simulink model "modelo_quad13_ver76"  (Simulink 8.3)
settings: Solver=ode45  StartTime=0.0  StopTime=100  FixedStep=0.025  MaxStep=0.1  RelTol=1e-3
values from neighbouring files (symbols this model uses):
  accel_noise = 0    [main_quad.m]
  baccx = 1e-1    (= 0.1)    [main_quad.m]
  baccy = 1e-1    (= 0.1)    [main_quad.m]
  baccz = 1e-1    (= 0.1)    [main_quad.m]
  baro_noise = 0    [main_quad.m]
  bgyrp = 1e-3    (= 0.001)    [main_quad.m]
  bgyrq = 1e-3    (= 0.001)    [main_quad.m]
  bgyrr = 1e-3    (= 0.001)    [main_quad.m]
  bmagx = 1e-6    (= 1e-06)    [main_quad.m]
  bmagy = -1e-6    (= -1e-06)    [main_quad.m]
  bmagz = 1e-6    (= 1e-06)    [main_quad.m]
  controle = 0    [main_quad.m]
  correct_acc = 1    [main_quad.m]
  cq = 2.4086*10^(-7)    (= 2.4086e-07)    [main_quad.m]
  cq_real = cq    (= 2.4086e-07)    [main_quad.m]
  ct = 1.4341*10^(-5)    (= 1.4341e-05)    [main_quad.m]
  ct_real = ct    (= 1.4341e-05)    [main_quad.m]
  d = 0.26    [main_quad.m]
  g = 9.8065    [main_quad.m]
  gps_noise_on = 0    [main_quad.m]
  gyro_noise = 0    [main_quad.m]
  J = [Jxx,Jyy,Jzz,Jm]    [main_quad.m]
  J_real = J    [main_quad.m]
  Ja = 5e-5    (= 5e-05)    [main_quad.m]
  k1 = 2.5    [main_quad.m]
  k2 = 6.2360    (= 6.236)    [main_quad.m]
  k3 = 6.2360    (= 6.236)    [main_quad.m]
  k4 = 0.4927    [main_quad.m]
  k5 = 1.6    [main_quad.m]
  k6 = 1.6    [main_quad.m]
  ke = kt    (= 0.024)    [main_quad.m]
  kt = 0.024    [main_quad.m]
  lambda1 = 1    [main_quad.m]
  lambda2 = 5    [main_quad.m]
  lambda3 = 5    [main_quad.m]
  lambda4 = 1/2    (= 0.5)    [main_quad.m]
  lambda5 = 1/4    (= 0.25)    [main_quad.m]
  lambda6 = 1/4    (= 0.25)    [main_quad.m]
  limit = [0.5 0.5 0.5 0.5]    [main_quad.m]
  limit_pos = [0.5 0.5]    [main_quad.m]
  m = 1.03    [main_quad.m]
  m_real = m    (= 1.03)    [main_quad.m]
  mag_noise = 0    [main_quad.m]
  max_w = 733.03    [main_quad.m]
  mgeo = [17223.7  -4581.6 -13698.2 ]'*1e-9    [main_quad.m]
  p0 = 0    [main_quad.m]
  phi0 = 0    [main_quad.m]
  Pitch_D = 0.019    [main_quad.m]
  Pitch_P = 0.019948    [main_quad.m]
  pos_D = -0.033991    [main_quad.m]
  pos_P = -0.005948    [main_quad.m]
  psi0 = 0    [main_quad.m]
  q0 = 0    [main_quad.m]
  R = 0.2    [main_quad.m]    (also in plot_resultados.m = A(:,12))
  r0 = 0    [main_quad.m]
  Roll_D = 0.019    [main_quad.m]
  Roll_P = 0.019948    [main_quad.m]
  t_d = 50e-3    (= 0.05)    [main_quad.m]
  theta0 = 0    [main_quad.m]
  Tnoise_gps = TsGPS    (= 0.2)    [main_quad.m]
  Ts_bar = 0.1    [main_quad.m]
  TsGPS = 1/fGPS    (= 0.2)    [main_quad.m]
  Tsr = 1e-2    (= 0.01)    [main_quad.m]
  vx0 = 0    [main_quad.m]
  vy0 = 0    [main_quad.m]
  vz0 = 0    [main_quad.m]
  w1_0 = w_hover    [main_quad.m]
  w2_0 = w_hover    [main_quad.m]
  w3_0 = w_hover    [main_quad.m]
  w4_0 = w_hover    [main_quad.m]
  w_f_gps = 2*pi*(2*fGPS)    (= 62.8318530718)    [main_quad.m]
  w_f_triad = 2*pi*(10)    (= 62.8318530718)    [main_quad.m]
  x0 = 0    [main_quad.m]
  y0 = 0    [main_quad.m]
  Yaw_D = 0.037200    (= 0.0372)    [main_quad.m]
  Yaw_P = 0.039055    [main_quad.m]
  z0 = 0    [main_quad.m]
  Z_D = -0.682000    (= -0.682)    [main_quad.m]
  Z_P = -0.238672    [main_quad.m]
libraries: simulink x18
(part 1 of 2)
settings Model: Creator=Germano  LastModifiedBy=andre
settings DataIOCC: LimitDataPoints=off
settings DebuggingCC: FcnCallInpInsideContextMsg=EnableAllAsWarning

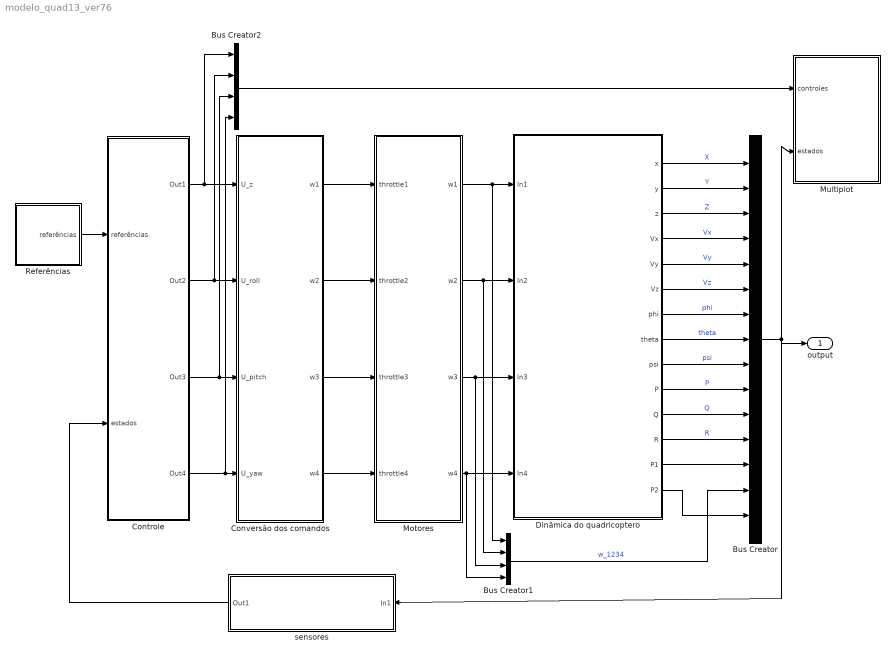
== system modelo_quad13_ver76 ==
  Bus Creator : BusCreator  Inputs=15
  Bus Creator1 : BusCreator
  Bus Creator2 : BusCreator
  Controle : Subsystem
  Conversão dos comandos : Subsystem
  Dinâmica do quadricoptero : Subsystem
  Motores : Subsystem
  Multiplot : Subsystem
  Referências : Subsystem
  sensores : Subsystem
  output : Outport
  wires:
  Bus Creator/1 -> sensores/1(In1), Multiplot/2(estados), output/1
  Motores/4(w4) -> Dinâmica do quadricoptero/4(In4), Bus Creator1/4
  Motores/1(w1) -> Bus Creator1/1, Dinâmica do quadricoptero/1(In1)
  Motores/3(w3) -> Dinâmica do quadricoptero/3(In3), Bus Creator1/3
  Motores/2(w2) -> Bus Creator1/2, Dinâmica do quadricoptero/2(In2)
  Conversão dos comandos/1(w1) -> Motores/1(throttle1)
  Conversão dos comandos/2(w2) -> Motores/2(throttle2)
  Conversão dos comandos/3(w3) -> Motores/3(throttle3)
  Conversão dos comandos/4(w4) -> Motores/4(throttle4)
  Dinâmica do quadricoptero/1(x) -> Bus Creator/1  "X"
  Dinâmica do quadricoptero/2(y) -> Bus Creator/2  "Y"
  Dinâmica do quadricoptero/3(z) -> Bus Creator/3  "Z"
  Dinâmica do quadricoptero/4(Vx) -> Bus Creator/4  "Vx"
  Dinâmica do quadricoptero/5(Vy) -> Bus Creator/5  "Vy"
  Dinâmica do quadricoptero/6(Vz) -> Bus Creator/6  "Vz"
  Dinâmica do quadricoptero/7(phi) -> Bus Creator/7  "phi"
  Dinâmica do quadricoptero/8(theta) -> Bus Creator/8  "theta"
  Dinâmica do quadricoptero/9(psi) -> Bus Creator/9  "psi"
  Dinâmica do quadricoptero/10(P) -> Bus Creator/10  "P"
  Dinâmica do quadricoptero/11(Q) -> Bus Creator/11  "Q"
  Dinâmica do quadricoptero/12(R) -> Bus Creator/12  "R"
  Controle/1(Out1) -> Bus Creator2/1, Conversão dos comandos/1(U_z)
  Controle/2(Out2) -> Bus Creator2/2, Conversão dos comandos/2(U_roll)
  Controle/3(Out3) -> Bus Creator2/3, Conversão dos comandos/3(U_pitch)
  Controle/4(Out4) -> Bus Creator2/4, Conversão dos comandos/4(U_yaw)
  Referências/1("referências ") -> Controle/1(referências)
  sensores/1(Out1) -> Controle/2(estados)
  Bus Creator2/1 -> Multiplot/1(controles)
  Dinâmica do quadricoptero/13(P1) -> Bus Creator/13
  Bus Creator1/1 -> Bus Creator/14  "w_1234"
  Dinâmica do quadricoptero/14(P2) -> Bus Creator/15

== system modelo_quad13_ver76/Controle ==
  note: 0: controle Sliding Mode
      | 1: controle PD
  referências : Inport
  estados : Inport  Port=2
  Constant : Constant  Value=controle
  Controlador PD : Subsystem
  Controlador sliding mode : Subsystem
  Demux : Demux
  Switch : Switch  Criteria=u2 > Threshold
  Out1 : Outport
  Out2 : Outport  Port=2
  Out3 : Outport  Port=3
  Out4 : Outport  Port=4
  wires:
  referências/1 -> Controlador sliding mode/1(Referências), Controlador PD/1(Referências)
  estados/1 -> Controlador sliding mode/2(Estados), Controlador PD/2(Estados)
  Switch/1 -> Demux/1
  Demux/1 -> Out1/1  "U_T"
  Demux/2 -> Out2/1  "U_L"
  Constant/1 -> Switch/2
  Demux/3 -> Out3/1  "U_M"
  Demux/4 -> Out4/1  "U_N"
  Controlador PD/1(Out1) -> Switch/1
  Controlador sliding mode/1(Out1) -> Switch/3

== system modelo_quad13_ver76/Conversão dos comandos ==
  U_z : Inport
  U_roll : Inport  Port=2
  U_pitch : Inport  Port=3
  U_yaw : Inport  Port=4
  Constant1 : Constant  Value=ct
  Constant2 : Constant  Value=cq
  Constant4 : Constant  Value=d
  MATLAB Function : MATLAB Function  TreatAsAtomicUnit=on
  w1 : Outport
  w2 : Outport  Port=2
  w3 : Outport  Port=3
  w4 : Outport  Port=4
  wires:
  U_pitch/1 -> MATLAB Function/3(u_M)
  U_z/1 -> MATLAB Function/1(u_T)
  U_yaw/1 -> MATLAB Function/4(u_N)
  Constant4/1 -> MATLAB Function/5(d)
  Constant1/1 -> MATLAB Function/6(ct)
  Constant2/1 -> MATLAB Function/7(cq)
  U_roll/1 -> MATLAB Function/2(u_L)
  MATLAB Function/1(w1d) -> w1/1  "w1d"
  MATLAB Function/2(w2d) -> w2/1  "w2d"
  MATLAB Function/3(w3d) -> w3/1  "w3d"
  MATLAB Function/4(w4d) -> w4/1  "w4d"

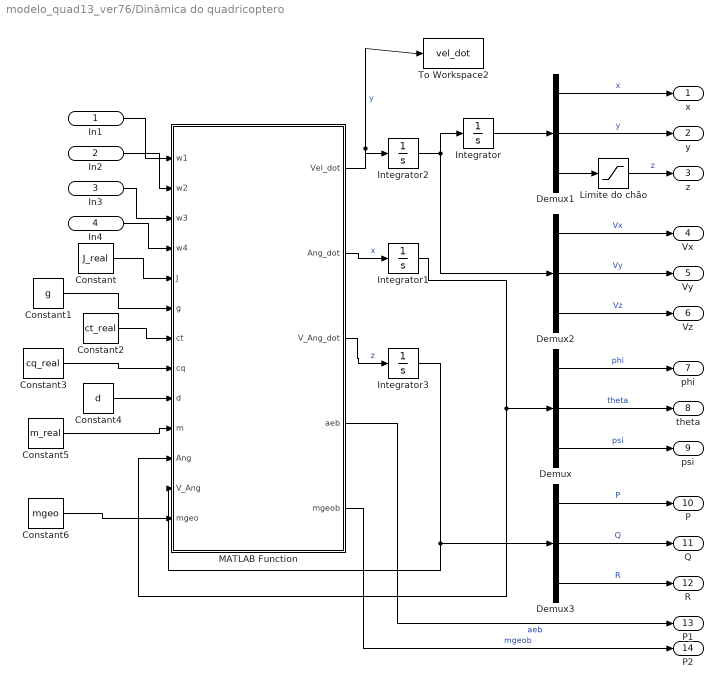
== system modelo_quad13_ver76/Dinâmica do quadricoptero ==
  In1 : Inport
  In2 : Inport  Port=2
  In3 : Inport  Port=3
  In4 : Inport  Port=4
  Constant : Constant  Value=J_real
  Constant1 : Constant  Value=g
  Constant2 : Constant  Value=ct_real
  Constant3 : Constant  Value=cq_real
  Constant4 : Constant  Value=d
  Constant5 : Constant  Value=m_real
  Constant6 : Constant  Value=mgeo
  Demux{,1..3} (4 alike) : Demux  Outputs=3
  Integrator : Integrator  InitialCondition=[x0;y0;z0]
  Integrator1 : Integrator  InitialCondition=[phi0;theta0;psi0]
  Integrator2 : Integrator  InitialCondition=[vx0;vy0;vz0;]
  Integrator3 : Integrator  InitialCondition=[p0;q0;r0]
  Limite do chão : Saturate  UpperLimit=0  LowerLimit=-Inf
  MATLAB Function : MATLAB Function  TreatAsAtomicUnit=on
  To Workspace2 : ToWorkspace  VariableName=vel_dot  SampleTime=-1
  x : Outport
  y : Outport  Port=2
  z : Outport  Port=3
  Vx : Outport  Port=4
  Vy : Outport  Port=5
  Vz : Outport  Port=6
  phi : Outport  Port=7
  theta : Outport  Port=8
  psi : Outport  Port=9
  P : Outport  Port=10
  Q : Outport  Port=11
  R : Outport  Port=12
  P1 : Outport  Port=13
  P2 : Outport  Port=14
  wires:
  In1/1 -> MATLAB Function/1(w1)
  In2/1 -> MATLAB Function/2(w2)
  In3/1 -> MATLAB Function/3(w3)
  In4/1 -> MATLAB Function/4(w4)
  Demux1/1 -> x/1  "x"
  Demux1/2 -> y/1  "y"
  Demux2/1 -> Vx/1  "Vx"
  Demux2/2 -> Vy/1  "Vy"
  Demux2/3 -> Vz/1  "Vz"
  MATLAB Function/1(Vel_dot) -> To Workspace2/1, Integrator2/1  "y"
  Integrator1/1 -> Demux/1, MATLAB Function/11(Ang)
  Demux/1 -> phi/1  "phi"
  Demux/2 -> theta/1  "theta"
  Demux/3 -> psi/1  "psi"
  MATLAB Function/2(Ang_dot) -> Integrator1/1  "x"
  Demux3/1 -> P/1  "P"
  Demux3/2 -> Q/1  "Q"
  Demux3/3 -> R/1  "R"
  MATLAB Function/3(V_Ang_dot) -> Integrator3/1  "z"
  Integrator2/1 -> Demux2/1, Integrator/1
  Integrator3/1 -> Demux3/1, MATLAB Function/12(V_Ang)
  Constant/1 -> MATLAB Function/5(J)
  Constant1/1 -> MATLAB Function/6(g)
  Constant2/1 -> MATLAB Function/7(ct)
  Constant3/1 -> MATLAB Function/8(cq)
  Constant4/1 -> MATLAB Function/9(d)
  Constant5/1 -> MATLAB Function/10(m)
  Integrator/1 -> Demux1/1
  Demux1/3 -> Limite do chão/1
  Limite do chão/1 -> z/1  "z"
  MATLAB Function/4(aeb) -> P1/1  "aeb"
  MATLAB Function/5(mgeob) -> P2/1  "mgeob"
  Constant6/1 -> MATLAB Function/13(mgeo)

== system modelo_quad13_ver76/Motores ==
  throttle1 : Inport
  throttle2 : Inport  Port=2
  throttle3 : Inport  Port=3
  throttle4 : Inport  Port=4
  Motor 1 : Subsystem
  Motor 2 : Subsystem
  Motor 3 : Subsystem
  Motor 4 : Subsystem
  w1 : Outport
  w2 : Outport  Port=2
  w3 : Outport  Port=3
  w4 : Outport  Port=4
  wires:
  throttle1/1 -> Motor 1/1(In1)  "w1d"
  throttle3/1 -> Motor 3/1(In1)  "w3d"
  throttle4/1 -> Motor 4/1(In1)  "w4d"
  throttle2/1 -> Motor 2/1(In1)  "w2d"
  Motor 1/1(Out1) -> w1/1  "w1"
  Motor 3/1(Out1) -> w3/1  "w3"
  Motor 4/1(Out1) -> w4/1  "w4"
  Motor 2/1(Out1) -> w2/1  "w2"

== system modelo_quad13_ver76/Multiplot ==
  controles : Inport
  estados : Inport  Port=2
  Bus Creator{1..4} (4 alike) : BusCreator  Inputs=3
  Bus Selector : BusSelector  OutputSignals=X,Y,Z,Vx,Vy,Vz,phi,theta,psi,P,Q,R,w_1234
  Gain : Gain  Gain=-1
  Gain1 : Gain  Gain=-1
  Gain2 : Gain  Gain=180/pi
  Gain3 : Gain  Gain=180/pi
  Gain4 : Gain  Gain=9.54929
  wires:
  estados/1 -> Bus Selector/1
  Bus Selector/2 -> Bus Creator2/2  "<Y>"
  Bus Selector/3 -> Gain/1  "<Z>"
  Bus Selector/1 -> Bus Creator2/1  "<X>"
  Bus Selector/6 -> Gain1/1  "<Vz>"
  Bus Selector/4 -> Bus Creator1/1  "<Vx>"
  Bus Selector/5 -> Bus Creator1/2  "<Vy>"
  Bus Selector/8 -> Bus Creator3/2  "<theta>"
  Bus Selector/7 -> Bus Creator3/1  "<phi>"
  Bus Selector/9 -> Bus Creator3/3  "<psi>"
  Bus Selector/11 -> Bus Creator4/2  "<Q>"
  Bus Selector/10 -> Bus Creator4/1  "<P>"
  Bus Selector/12 -> Bus Creator4/3  "<R>"
  Bus Creator2/1 -> ?
  Bus Creator1/1 -> ?
  controles/1 -> ?
  Gain/1 -> Bus Creator2/3
  Gain1/1 -> Bus Creator1/3
  Bus Creator3/1 -> Gain2/1
  Gain2/1 -> ?
  Bus Creator4/1 -> Gain3/1
  Gain3/1 -> ?
  Bus Selector/13 -> Gain4/1  "<w_1234>"
  Gain4/1 -> ?

== system modelo_quad13_ver76/Referências ==
  Gain1 : Gain
  Gain2 : Gain
  Gain3 : Gain  Gain=-1
  Gain4 : Gain
  Mux : Mux
  Step1 : Step  Time=75  After=15*pi/180  SampleTime=0
  Step2 : Step  Time=5  After=10  SampleTime=0
  Step_x : Step  Time=10  After=10  SampleTime=0
  Step_y : Step  Time=30  After=10  SampleTime=0
  "referências " : Outport
  wires:
  Mux/1 -> "referências "/1
  Gain3/1 -> Mux/3  "ref_z"
  Step_y/1 -> Gain2/1
  Gain2/1 -> Mux/2  "ref_y"
  Step_x/1 -> Gain4/1
  Gain4/1 -> Mux/1  "ref_x"
  Gain1/1 -> Mux/4  "ref_psi"
  Step2/1 -> Gain3/1
  Step1/1 -> Gain1/1

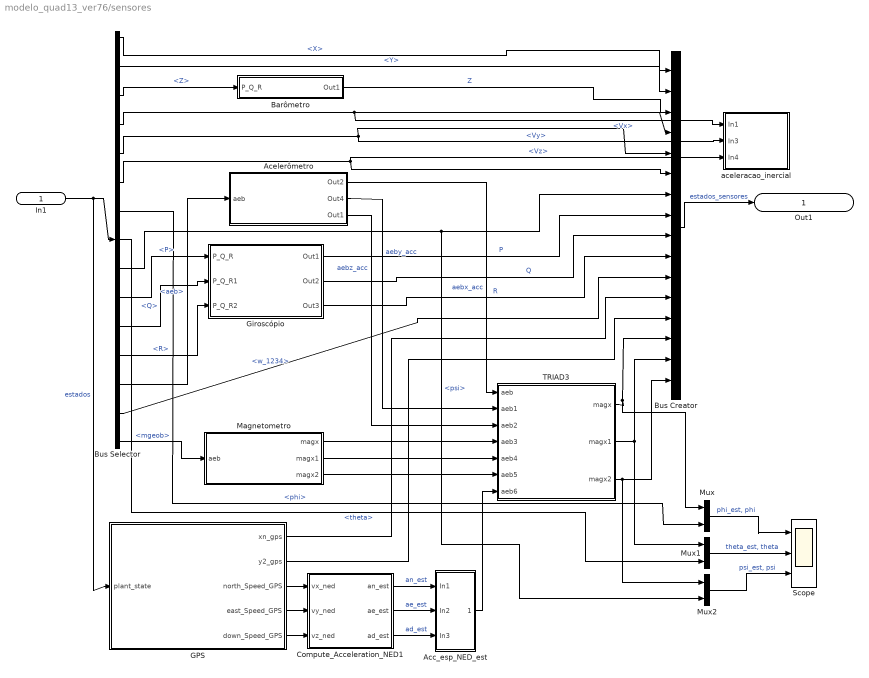
== system modelo_quad13_ver76/sensores ==
  In1 : Inport
  Acc_esp_NED_est : Subsystem
  Acelerômetro : Subsystem
  Barômetro : Subsystem
  Bus Creator : BusCreator  Inputs=16
  Bus Selector : BusSelector  OutputSignals=X,Y,Z,Vx,Vy,Vz,phi,theta,psi,P,Q,R,aeb,w_1234,mgeob
  Compute_Acceleration_NED1 : Subsystem
  GPS : Subsystem
  Giroscópio : Subsystem
  Magnetometro : Subsystem
  Mux : Mux  Inputs=2
  Mux1 : Mux  Inputs=2
  Mux2 : Mux  Inputs=2
  Scope : Scope  NumInputPorts=3
      settings: YMin=-2.5~-1.5~-1.75  YMax=2~0.25~1.75  SaveName=ScopeData8
  TRIAD3 : Subsystem
  aceleracao_inercial : Subsystem
  Out1 : Outport
  wires:
  In1/1 -> Bus Selector/1, GPS/1(plant_state)  "estados"
  Bus Selector/4 -> Bus Creator/4, aceleracao_inercial/1(In1)  "<Vx>"
  Bus Selector/6 -> Bus Creator/6, aceleracao_inercial/3(In4)  "<Vz>"
  Bus Selector/1 -> Bus Creator/1  "<X>"
  Bus Selector/3 -> Barômetro/1(P_Q_R)  "<Z>"
  Bus Selector/2 -> Bus Creator/2  "<Y>"
  Bus Selector/5 -> Bus Creator/5, aceleracao_inercial/2(In3)  "<Vy>"
  Bus Creator/1 -> Out1/1  "estados_sensores"
  Bus Selector/10 -> Giroscópio/1(P_Q_R)  "<P>"
  Bus Selector/11 -> Giroscópio/2(P_Q_R1)  "<Q>"
  Bus Selector/12 -> Giroscópio/3(P_Q_R2)  "<R>"
  Giroscópio/3(Out3) -> Bus Creator/10  "R"
  Giroscópio/2(Out2) -> Bus Creator/9  "Q"
  Giroscópio/1(Out1) -> Bus Creator/8  "P"
  Bus Selector/14 -> Bus Creator/11  "<w_1234>"
  Bus Selector/9 -> Bus Creator/7, Mux2/2  "<psi>"
  Bus Selector/13 -> Acelerômetro/1(aeb)  "<aeb>"
  Bus Selector/15 -> Magnetometro/1(aeb)  "<mgeob>"
  Acelerômetro/1(Out2) -> TRIAD3/1(aeb)  "aebx_acc"
  Acelerômetro/2(Out4) -> TRIAD3/2(aeb1)  "aeby_acc"
  Acelerômetro/3(Out1) -> TRIAD3/3(aeb2)  "aebz_acc"
  Magnetometro/1(magx) -> TRIAD3/4(aeb3)
  Magnetometro/2(magx1) -> TRIAD3/5(aeb4)
  Magnetometro/3(magx2) -> TRIAD3/6(aeb5)
  GPS/2(y2_gps) -> Bus Creator/13
  GPS/3(north_Speed_GPS) -> Compute_Acceleration_NED1/1(vx_ned)
  GPS/4(east_Speed_GPS) -> Compute_Acceleration_NED1/2(vy_ned)
  GPS/5(down_Speed_GPS) -> Compute_Acceleration_NED1/3(vz_ned)
  Compute_Acceleration_NED1/1(an_est) -> Acc_esp_NED_est/1(In1)  "an_est"
  Compute_Acceleration_NED1/2(ae_est) -> Acc_esp_NED_est/2(In2)  "ae_est"
  Compute_Acceleration_NED1/3(ad_est) -> Acc_esp_NED_est/3(In3)  "ad_est"
  Acc_esp_NED_est/1(Out1) -> TRIAD3/7(aeb6)
  GPS/1(xn_gps) -> Bus Creator/12
  Barômetro/1(Out1) -> Bus Creator/3  "Z"
  TRIAD3/1(magx) -> Bus Creator/14, Mux/1
  TRIAD3/2(magx1) -> Bus Creator/15, Mux1/1
  TRIAD3/3(magx2) -> Bus Creator/16, Mux2/1
  Mux/1 -> Scope/1  "phi_est, phi"
  Mux1/1 -> Scope/2  "theta_est, theta"
  Mux2/1 -> Scope/3  "psi_est, psi"
  Bus Selector/8 -> Mux1/2  "<theta>"
  Bus Selector/7 -> Mux/2  "<phi>"

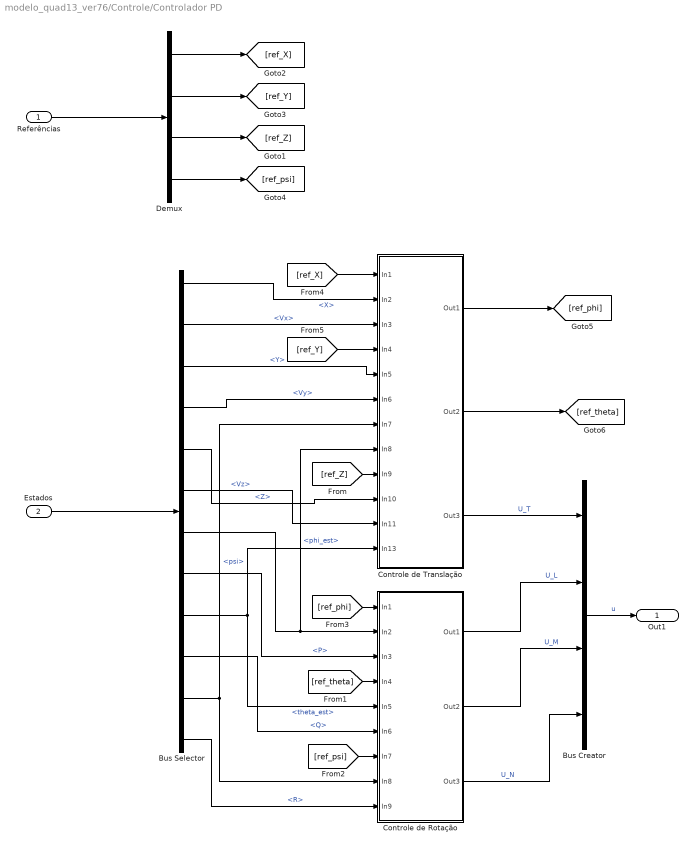
== system modelo_quad13_ver76/Controle/Controlador PD ==
  Referências : Inport
  Estados : Inport  Port=2
  Bus Creator : BusCreator
  Bus Selector : BusSelector  OutputSignals=X,Vx,Y,Vy,Z,Vz,phi_est,P,theta_est,Q,psi,R
  Controle de Rotação : Subsystem
  Controle de Translação : Subsystem
  Demux : Demux
  Out1 : Outport
  wires:
  Demux/4 -> [ref_psi]
  Bus Creator/1 -> Out1/1  "u"
  Demux/1 -> [ref_X]
  Demux/2 -> [ref_Y]
  Demux/3 -> [ref_Z]
  [ref_phi] -> Controle de Rotação/1(In1)
  [ref_theta] -> Controle de Rotação/4(In4)
  Controle de Rotação/1(Out1) -> Bus Creator/2  "U_L"
  Controle de Rotação/2(Out2) -> Bus Creator/3  "U_M"
  Controle de Rotação/3(Out3) -> Bus Creator/4  "U_N"
  [ref_X] -> Controle de Translação/1(In1)
  Controle de Translação/3(Out3) -> Bus Creator/1  "U_T"
  [ref_Y] -> Controle de Translação/4(In4)
  [ref_Z] -> Controle de Translação/9(In9)
  Bus Selector/1 -> Controle de Translação/2(In2)  "<X>"
  Bus Selector/2 -> Controle de Translação/3(In3)  "<Vx>"
  Bus Selector/3 -> Controle de Translação/5(In5)  "<Y>"
  Bus Selector/4 -> Controle de Translação/6(In6)  "<Vy>"
  Bus Selector/5 -> Controle de Translação/10(In10)  "<Z>"
  Bus Selector/6 -> Controle de Translação/11(In11)  "<Vz>"
  Bus Selector/7 -> Controle de Translação/8(In8), Controle de Rotação/2(In2)  "<phi_est>"
  Bus Selector/8 -> Controle de Rotação/3(In3)  "<P>"
  Bus Selector/9 -> Controle de Rotação/5(In5), Controle de Translação/12(In13)  "<theta_est>"
  Bus Selector/10 -> Controle de Rotação/6(In6)  "<Q>"
  Bus Selector/11 -> Controle de Rotação/8(In8), Controle de Translação/7(In7)  "<psi>"
  Bus Selector/12 -> Controle de Rotação/9(In9)  "<R>"
  [ref_psi] -> Controle de Rotação/7(In7)
  Referências/1 -> Demux/1
  Estados/1 -> Bus Selector/1
  Controle de Translação/1(Out1) -> [ref_phi]
  Controle de Translação/2(Out2) -> [ref_theta]

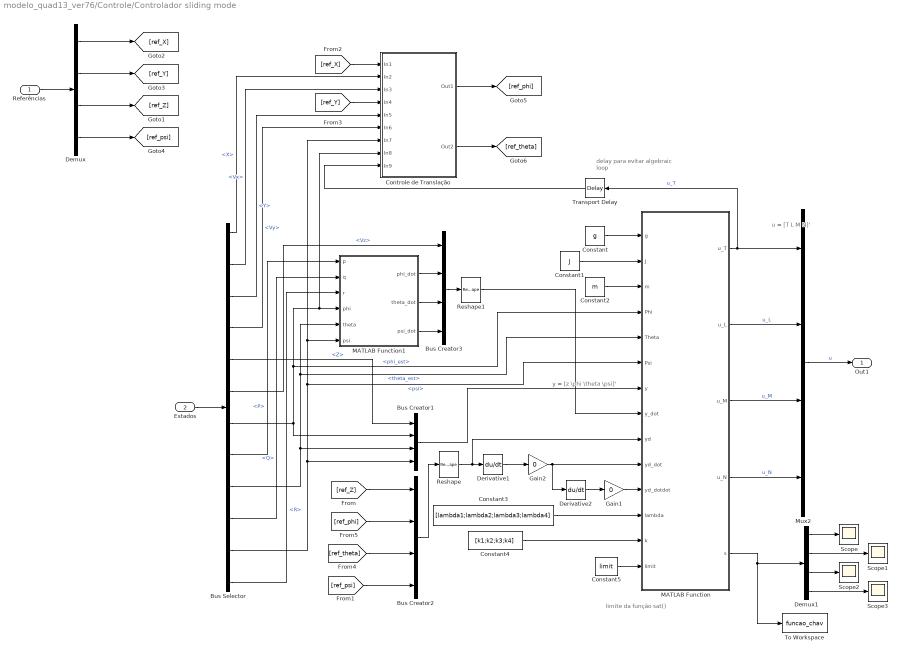
== system modelo_quad13_ver76/Controle/Controlador sliding mode ==
  note: limite da função sat()
  note: delay para evitar
      |  algebraic loop
  note: y = [z \phi \theta \psi]'
  note: u = [T L M N]'
  Referências : Inport
  Estados : Inport  Port=2
  Bus Creator1 : BusCreator
  Bus Creator2 : BusCreator
  Bus Creator3 : BusCreator
  Bus Selector : BusSelector  OutputSignals=X,Vx,Y,Vy,Z,Vz,phi_est,P,theta_est,Q,psi,R
  Constant : Constant  Value=g
  Constant1 : Constant  Value=J
  Constant2 : Constant  Value=m
  Constant3 : Constant  Value=[lambda1;lambda2;lambda3;lambda4]
  Constant4 : Constant  Value=[k1;k2;k3;k4]
  Constant5 : Constant  Value=limit
  Controle de Translação : Subsystem
  Demux : Demux
  Demux1 : Demux
  Derivative1 : Derivative
  Derivative2 : Derivative
  Gain1 : Gain  Gain=0
  Gain2 : Gain  Gain=0
  MATLAB Function : MATLAB Function  TreatAsAtomicUnit=on
  MATLAB Function1 : MATLAB Function  TreatAsAtomicUnit=on
  Mux2 : Mux
  Reshape : Reshape  OutputDimensionality=Customize  OutputDimensions=[4,1]
  Reshape1 : Reshape  OutputDimensionality=Customize  OutputDimensions=[4,1]
  Scope{,1..3} (4 alike) : Scope
      Scope settings: TimeRange=100  YMin=-1
      Scope1 settings: TimeRange=100  YMin=-1  SaveName=ScopeData4
      Scope2 settings: TimeRange=100  YMin=-1  SaveName=ScopeData5
      Scope3 settings: TimeRange=100  YMin=-1  SaveName=ScopeData6
  To Workspace : ToWorkspace  VariableName=funcao_chav  SampleTime=-1
  Transport Delay : TransportDelay  DelayTime=0.01  InitialOutput=m*g
  Out1 : Outport
  wires:
  Demux/4 -> [ref_psi]
  Estados/1 -> Bus Selector/1
  Referências/1 -> Demux/1
  Demux/1 -> [ref_X]
  Demux/2 -> [ref_Y]
  Demux/3 -> [ref_Z]
  Constant/1 -> MATLAB Function/1(g)
  Constant1/1 -> MATLAB Function/2(J)
  Constant2/1 -> MATLAB Function/3(m)
  Bus Selector/5 -> Bus Creator1/1  "<Z>"
  Bus Selector/7 -> Bus Creator1/2, MATLAB Function/4(Phi), Controle de Translação/8(In8), MATLAB Function1/4(phi)  "<phi_est>"
  Bus Selector/9 -> Bus Creator1/3, MATLAB Function/5(Theta), MATLAB Function1/5(theta)  "<theta_est>"
  Bus Selector/11 -> Bus Creator1/4, Controle de Translação/7(In7), MATLAB Function1/6(psi), MATLAB Function/6(Psi)  "<psi>"
  Constant3/1 -> MATLAB Function/12(lambda)
  Bus Selector/8 -> MATLAB Function1/1(p)  "<P>"
  Bus Selector/10 -> MATLAB Function1/2(q)  "<Q>"
  Bus Selector/12 -> MATLAB Function1/3(r)  "<R>"
  Constant4/1 -> MATLAB Function/13(k)
  Derivative2/1 -> Gain1/1
  Mux2/1 -> Out1/1  "u"
  MATLAB Function/1(u_T) -> Mux2/1, Transport Delay/1  "u_T"
  MATLAB Function/2(u_L) -> Mux2/2  "u_L"
  MATLAB Function/4(u_N) -> Mux2/4  "u_N"
  MATLAB Function/3(u_M) -> Mux2/3  "u_M"
  Gain1/1 -> MATLAB Function/11(yd_dotdot)
  Gain2/1 -> Derivative2/1, MATLAB Function/10(yd_dot)
  Bus Selector/1 -> Controle de Translação/2(In2)  "<X>"
  Bus Selector/2 -> Controle de Translação/3(In3)  "<Vx>"
  Bus Selector/3 -> Controle de Translação/5(In5)  "<Y>"
  Bus Selector/4 -> Controle de Translação/6(In6)  "<Vy>"
  [ref_X] -> Controle de Translação/1(In1)
  [ref_Y] -> Controle de Translação/4(In4)
  [ref_Z] -> Bus Creator2/1
  [ref_psi] -> Bus Creator2/4
  Bus Creator2/1 -> Reshape/1
  [ref_theta] -> Bus Creator2/3
  [ref_phi] -> Bus Creator2/2
  Bus Creator1/1 -> MATLAB Function/7(y)
  Controle de Translação/1(Out1) -> [ref_phi]
  Controle de Translação/2(Out2) -> [ref_theta]
  Reshape/1 -> MATLAB Function/9(yd), Derivative1/1
  Transport Delay/1 -> Controle de Translação/9(In9)
  Constant5/1 -> MATLAB Function/14(limit)
  Bus Selector/6 -> Bus Creator3/1  "<Vz>"
  MATLAB Function1/1(phi_dot) -> Bus Creator3/2
  MATLAB Function1/2(theta_dot) -> Bus Creator3/3
  MATLAB Function1/3(psi_dot) -> Bus Creator3/4
  Bus Creator3/1 -> Reshape1/1
  Reshape1/1 -> MATLAB Function/8(y_dot)
  MATLAB Function/5(s) -> Demux1/1, To Workspace/1
  Derivative1/1 -> Gain2/1
  Demux1/1 -> Scope/1
  Demux1/2 -> Scope1/1
  Demux1/3 -> Scope2/1
  Demux1/4 -> Scope3/1

== system modelo_quad13_ver76/Motores/Motor 1 ==
  In1 : Inport
  Constant : Constant  Value=ke
  Constant1 : Constant  Value=cq
  Constant2 : Constant  Value=kt
  Constant3 : Constant  Value=R
  Constant4 : Constant  Value=Ja
  Integrator : Integrator  InitialCondition=w1_0
  MATLAB Function : MATLAB Function  TreatAsAtomicUnit=on
  Saturation : Saturate  UpperLimit=max_w  LowerLimit=0
  Out1 : Outport
  wires:
  MATLAB Function/1(wder) -> Integrator/1
  Saturation/1 -> MATLAB Function/2(w), Out1/1  "w1"
  Integrator/1 -> Saturation/1
  Constant/1 -> MATLAB Function/3(ke)
  Constant1/1 -> MATLAB Function/4(cq)
  Constant2/1 -> MATLAB Function/5(kt)
  Constant3/1 -> MATLAB Function/6(R)
  Constant4/1 -> MATLAB Function/7(Ja)
  In1/1 -> MATLAB Function/1(wd)

== system modelo_quad13_ver76/Motores/Motor 2 ==
  In1 : Inport
  Constant : Constant  Value=ke
  Constant1 : Constant  Value=cq
  Constant2 : Constant  Value=kt
  Constant3 : Constant  Value=R
  Constant4 : Constant  Value=Ja
  Integrator : Integrator  InitialCondition=w2_0
  MATLAB Function : MATLAB Function  TreatAsAtomicUnit=on
  Saturation : Saturate  UpperLimit=max_w  LowerLimit=0
  Out1 : Outport
  wires:
  MATLAB Function/1(wder) -> Integrator/1
  Saturation/1 -> MATLAB Function/2(w), Out1/1  "w2"
  Integrator/1 -> Saturation/1
  Constant/1 -> MATLAB Function/3(ke)
  Constant1/1 -> MATLAB Function/4(cq)
  Constant2/1 -> MATLAB Function/5(kt)
  Constant3/1 -> MATLAB Function/6(R)
  Constant4/1 -> MATLAB Function/7(Ja)
  In1/1 -> MATLAB Function/1(wd)

== system modelo_quad13_ver76/Motores/Motor 3 ==
  In1 : Inport
  Constant : Constant  Value=ke
  Constant1 : Constant  Value=cq
  Constant2 : Constant  Value=kt
  Constant3 : Constant  Value=R
  Constant4 : Constant  Value=Ja
  Integrator : Integrator  InitialCondition=w3_0
  MATLAB Function : MATLAB Function  TreatAsAtomicUnit=on
  Saturation : Saturate  UpperLimit=max_w  LowerLimit=0
  Out1 : Outport
  wires:
  MATLAB Function/1(wder) -> Integrator/1
  Saturation/1 -> MATLAB Function/2(w), Out1/1  "w3"
  Integrator/1 -> Saturation/1
  Constant/1 -> MATLAB Function/3(ke)
  Constant1/1 -> MATLAB Function/4(cq)
  Constant2/1 -> MATLAB Function/5(kt)
  Constant3/1 -> MATLAB Function/6(R)
  Constant4/1 -> MATLAB Function/7(Ja)
  In1/1 -> MATLAB Function/1(wd)

== system modelo_quad13_ver76/Motores/Motor 4 ==
  In1 : Inport
  Constant : Constant  Value=ke
  Constant1 : Constant  Value=cq
  Constant2 : Constant  Value=kt
  Constant3 : Constant  Value=R
  Constant4 : Constant  Value=Ja
  Integrator : Integrator  InitialCondition=w4_0
  MATLAB Function : MATLAB Function  TreatAsAtomicUnit=on
  Saturation : Saturate  UpperLimit=max_w  LowerLimit=0
  Out1 : Outport
  wires:
  MATLAB Function/1(wder) -> Integrator/1
  Saturation/1 -> MATLAB Function/2(w), Out1/1  "w4"
  Integrator/1 -> Saturation/1
  Constant/1 -> MATLAB Function/3(ke)
  Constant1/1 -> MATLAB Function/4(cq)
  Constant2/1 -> MATLAB Function/5(kt)
  Constant3/1 -> MATLAB Function/6(R)
  Constant4/1 -> MATLAB Function/7(Ja)
  In1/1 -> MATLAB Function/1(wd)

== system modelo_quad13_ver76/sensores/Acc_esp_NED_est ==
  In1 : Inport
  In2 : Inport  Port=2
  In3 : Inport  Port=3
  Add : Sum  Inputs=+-
  Gain : Gain  Gain=correct_acc
  Mux2 : Mux  Inputs=3
  acc_grav_ned : Constant  Value=[0 0 g]'
  Out1 : Outport
  wires:
  Mux2/1 -> Gain/1  "acc_ned_est"
  acc_grav_ned/1 -> Add/2
  In1/1 -> Mux2/1  "an_ned"
  In2/1 -> Mux2/2  "ae_ned"
  Add/1 -> Out1/1  "a_esp_ned"
  In3/1 -> Mux2/3  "ad_ned"
  Gain/1 -> Add/1

== system modelo_quad13_ver76/sensores/Acelerômetro ==
  aeb : Inport
  Demux : Demux  Outputs=3
  Inclusão ruídos : Subsystem
  Scope1 : Scope  NumInputPorts=3
      settings: YMin=-0.75~-0.75~-10.75  YMax=1~1~-8.75  SaveName=ScopeData9
  Out2 : Outport
  Out4 : Outport  Port=2
  Out1 : Outport  Port=3
  wires:
  aeb/1 -> Demux/1  "aeb"
  Demux/2 -> Inclusão ruídos/2(P_Q_R1)
  Demux/3 -> Inclusão ruídos/3(P_Q_R2)
  Demux/1 -> Inclusão ruídos/1(P_Q_R)
  Inclusão ruídos/1(Out1) -> Out2/1, Scope1/1  "aebx_acc"
  Inclusão ruídos/2(Out2) -> Out4/1, Scope1/2  "aeby_acc"
  Inclusão ruídos/3(Out3) -> Out1/1, Scope1/3  "aebz_acc"

== system modelo_quad13_ver76/sensores/Barômetro ==
  P_Q_R : Inport
  Add3 : Sum
  Band-Limited White Noise : simulink/Sources/Band-Limited White Noise  Cov=varbar  Ts=Ts_bar  seed=[23341]
  Gain : Gain  Gain=baro_noise
  Scope : Scope
      settings: YMin=-13  YMax=3  SaveName=ScopeData12
  Out1 : Outport
  wires:
  Add3/1 -> Out1/1, Scope/1  "z_baro"
  P_Q_R/1 -> Add3/1  "z"
  Band-Limited White Noise/1 -> Gain/1
  Gain/1 -> Add3/2

== system modelo_quad13_ver76/sensores/Compute_Acceleration_NED1 ==
  vx_ned : Inport
  vy_ned : Inport  Port=2
  vz_ned : Inport  Port=3
  Scope : Scope  NumInputPorts=3
      settings: YMin=-1~-1~-2.5  YMax=1~1~0
  Scope1 : Scope  NumInputPorts=3
      settings: YMin=-50~-75~-125  YMax=50~75~100  SaveName=ScopeData2
  Transfer Fcn : TransferFcn  Numerator=[1 0]  Denominator=[t_d 1]
  Transfer Fcn1 : TransferFcn  Numerator=[1 0]  Denominator=[t_d 1]
  Transfer Fcn2 : TransferFcn  Numerator=[1 0]  Denominator=[t_d 1]
  Transfer Fcn3 : TransferFcn  Numerator=[w_f_gps]  Denominator=[1 w_f_gps]
  Transfer Fcn4 : TransferFcn  Numerator=[w_f_gps]  Denominator=[1 w_f_gps]
  Transfer Fcn5 : TransferFcn  Numerator=[w_f_gps]  Denominator=[1 w_f_gps]
  an_est : Outport
  ae_est : Outport  Port=2
  ad_est : Outport  Port=3
  wires:
  vy_ned/1 -> Transfer Fcn4/1
  vx_ned/1 -> Transfer Fcn3/1
  vz_ned/1 -> Transfer Fcn5/1
  Transfer Fcn/1 -> an_est/1, Scope1/1
  Transfer Fcn1/1 -> ae_est/1, Scope1/2
  Transfer Fcn2/1 -> ad_est/1, Scope1/3
  Transfer Fcn3/1 -> Scope/1, Transfer Fcn/1
  Transfer Fcn4/1 -> Scope/2, Transfer Fcn1/1
  Transfer Fcn5/1 -> Scope/3, Transfer Fcn2/1

== system modelo_quad13_ver76/sensores/GPS ==
  plant_state : Inport
  Bus Selector : BusSelector  OutputSignals=X,Y,Vx,Vy,Vz
  GPS_LAT : Subsystem
  GPS_LON : Subsystem
  GPS_VEL : Subsystem
  GPS_VEL1 : Subsystem
  GPS_VEL2 : Subsystem
  Scope1 : Scope  NumInputPorts=5
      settings: TimeRange=100  YMin=-2.5~-2.5~-1~-3~-5  YMax=12.5~12.5~3~3~2  SaveName=ScopeData13
  xn_gps : Outport
  y2_gps : Outport  Port=2
  north_Speed_GPS : Outport  Port=3
  east_Speed_GPS : Outport  Port=4
  down_Speed_GPS : Outport  Port=5
  wires:
  GPS_LON/1(ye_gps) -> y2_gps/1, Scope1/2
  Bus Selector/2 -> GPS_LON/1(east_Disp_m)  "<Y>"
  GPS_VEL1/1(east_Speed_GPS_mps) -> east_Speed_GPS/1, Scope1/4
  GPS_LAT/1(xn_gps) -> xn_gps/1, Scope1/1
  Bus Selector/1 -> GPS_LAT/1(north_Disp_m)  "<X>"
  GPS_VEL/1(north_Speed_GPS_mps) -> north_Speed_GPS/1, Scope1/3
  plant_state/1 -> Bus Selector/1
  Bus Selector/3 -> GPS_VEL/1(north_Speed_mps)  "<Vx>"
  Bus Selector/4 -> GPS_VEL1/1(east_Speed_mps)  "<Vy>"
  Bus Selector/5 -> GPS_VEL2/1(down_Speed_mps)  "<Vz>"
  GPS_VEL2/1(down_Speed_GPS_mps) -> down_Speed_GPS/1, Scope1/5

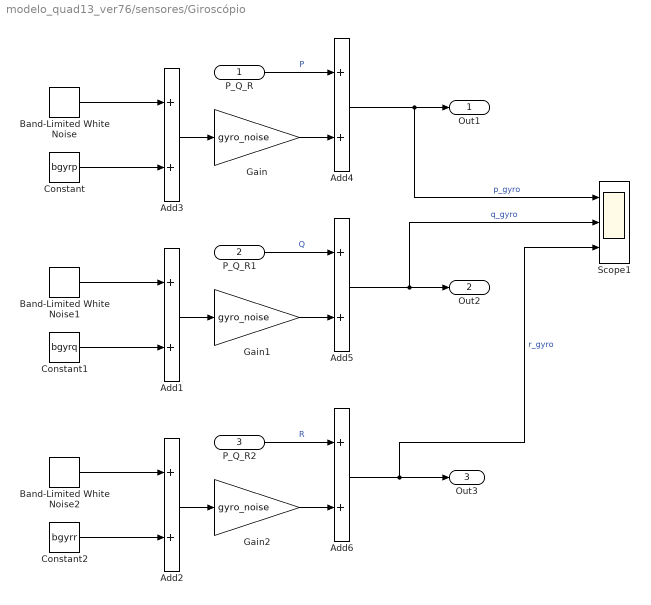
== system modelo_quad13_ver76/sensores/Giroscópio ==
  P_Q_R : Inport
  P_Q_R1 : Inport  Port=2
  P_Q_R2 : Inport  Port=3
  Add{1..6} (6 alike) : Sum
  Band-Limited White Noise : simulink/Sources/Band-Limited White Noise  Cov=varGyrp  Ts=Tsr  seed=[23341]
  Band-Limited White Noise1 : simulink/Sources/Band-Limited White Noise  Cov=varGyrq  Ts=Tsr  seed=[23341]
  Band-Limited White Noise2 : simulink/Sources/Band-Limited White Noise  Cov=varGyrr  Ts=Tsr  seed=[23341]
  Constant : Constant  Value=bgyrp
  Constant1 : Constant  Value=bgyrq
  Constant2 : Constant  Value=bgyrr
  Gain : Gain  Gain=gyro_noise
  Gain1 : Gain  Gain=gyro_noise
  Gain2 : Gain  Gain=gyro_noise
  Scope1 : Scope  NumInputPorts=3
      settings: YMin=-0.35~-0.3~-0.35  YMax=0.4~0.2~0.3  SaveName=ScopeData10
  Out1 : Outport
  Out2 : Outport  Port=2
  Out3 : Outport  Port=3
  wires:
  Constant/1 -> Add3/2
  Band-Limited White Noise/1 -> Add3/1
  Add3/1 -> Gain/1
  Gain/1 -> Add4/2
  P_Q_R/1 -> Add4/1  "P"
  Add4/1 -> Out1/1, Scope1/1  "p_gyro"
  Add5/1 -> Out2/1, Scope1/2  "q_gyro"
  Add1/1 -> Gain1/1
  Gain1/1 -> Add5/2
  P_Q_R1/1 -> Add5/1  "Q"
  Constant1/1 -> Add1/2
  Band-Limited White Noise1/1 -> Add1/1
  Add6/1 -> Out3/1, Scope1/3  "r_gyro"
  Add2/1 -> Gain2/1
  Gain2/1 -> Add6/2
  P_Q_R2/1 -> Add6/1  "R"
  Band-Limited White Noise2/1 -> Add2/1
  Constant2/1 -> Add2/2

== system modelo_quad13_ver76/sensores/Magnetometro ==
  aeb : Inport
  Demux : Demux  Outputs=3
  Inclusão ruídos : Subsystem
  Scope1 : Scope  NumInputPorts=3
      settings: YMin=2.1e-05~-1.2e-05~2.6e-05  YMax=3.3e-05~2e-06~3.7e-05  SaveName=ScopeData11
  magx : Outport
  magx1 : Outport  Port=2
  magx2 : Outport  Port=3
  wires:
  aeb/1 -> Demux/1  "mgeob"
  Demux/2 -> Inclusão ruídos/2(P_Q_R1)
  Demux/3 -> Inclusão ruídos/3(P_Q_R2)
  Demux/1 -> Inclusão ruídos/1(P_Q_R)
  Inclusão ruídos/1(Out1) -> magx/1, Scope1/1  "magx"
  Inclusão ruídos/2(Out2) -> magx1/1, Scope1/2  "magy"
  Inclusão ruídos/3(Out3) -> magx2/1, Scope1/3  "magz"

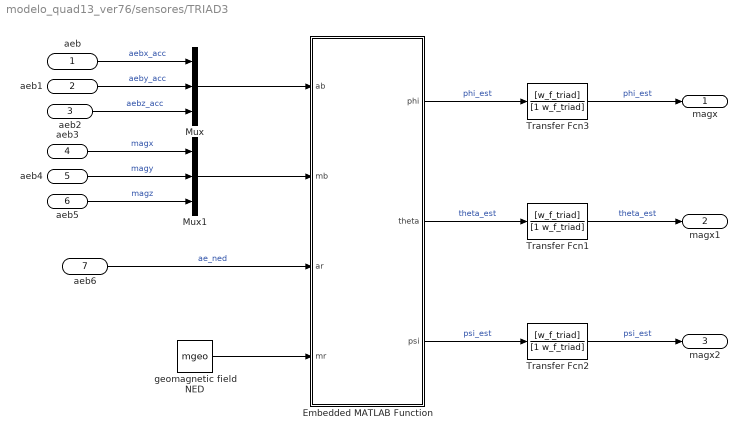
== system modelo_quad13_ver76/sensores/TRIAD3 ==
  aeb : Inport
  aeb1 : Inport  Port=2
  aeb2 : Inport  Port=3
  aeb3 : Inport  Port=4
  aeb4 : Inport  Port=5
  aeb5 : Inport  Port=6
  aeb6 : Inport  Port=7
  Embedded MATLAB Function : MATLAB Function  TreatAsAtomicUnit=on
  Mux : Mux  Inputs=3
  Mux1 : Mux  Inputs=3
  Transfer Fcn1 : TransferFcn  Numerator=[w_f_triad]  Denominator=[1 w_f_triad]
  Transfer Fcn2 : TransferFcn  Numerator=[w_f_triad]  Denominator=[1 w_f_triad]
  Transfer Fcn3 : TransferFcn  Numerator=[w_f_triad]  Denominator=[1 w_f_triad]
  geomagnetic field NED : Constant  Value=mgeo
  magx : Outport
  magx1 : Outport  Port=2
  magx2 : Outport  Port=3
  wires:
  aeb/1 -> Mux/1  "aebx_acc"
  aeb1/1 -> Mux/2  "aeby_acc"
  aeb2/1 -> Mux/3  "aebz_acc"
  Mux/1 -> Embedded MATLAB Function/1(ab)
  aeb3/1 -> Mux1/1  "magx"
  aeb4/1 -> Mux1/2  "magy"
  aeb5/1 -> Mux1/3  "magz"
  Mux1/1 -> Embedded MATLAB Function/2(mb)
  geomagnetic field NED/1 -> Embedded MATLAB Function/4(mr)
  aeb6/1 -> Embedded MATLAB Function/3(ar)  "ae_ned"
  Embedded MATLAB Function/1(phi) -> Transfer Fcn3/1  "phi_est"
  Embedded MATLAB Function/2(theta) -> Transfer Fcn1/1  "theta_est"
  Embedded MATLAB Function/3(psi) -> Transfer Fcn2/1  "psi_est"
  Transfer Fcn3/1 -> magx/1  "phi_est"
  Transfer Fcn1/1 -> magx1/1  "theta_est"
  Transfer Fcn2/1 -> magx2/1  "psi_est"

== system modelo_quad13_ver76/sensores/aceleracao_inercial ==
  In1 : Inport
  In3 : Inport  Port=2
  In4 : Inport  Port=3
  Derivative : Derivative
  Derivative1 : Derivative
  Derivative2 : Derivative
  Modulus : Subsystem
  Mux : Mux  Inputs=3
  Scope : Scope  NumInputPorts=4
      settings: YMin=-1~-1~-2.5~0  YMax=1.75~2~2~2.5  SaveName=ScopeData7
  wires:
  Derivative/1 -> Scope/1, Mux/1  "A_x"
  Derivative1/1 -> Scope/2, Mux/2  "A_y"
  Derivative2/1 -> Scope/3, Mux/3  "A_z"
  In1/1 -> Derivative/1
  In3/1 -> Derivative1/1
  In4/1 -> Derivative2/1
  Modulus/1(Out1) -> Scope/4
  Mux/1 -> Modulus/1(In1)

== system modelo_quad13_ver76/Controle/Controlador PD/Controle de Rotação ==
  In1 : Inport
  In2 : Inport  Port=2
  In3 : Inport  Port=3
  In4 : Inport  Port=4
  In5 : Inport  Port=5
  In6 : Inport  Port=6
  In7 : Inport  Port=7
  In8 : Inport  Port=8
  In9 : Inport  Port=9
  Controle de Pitch : Subsystem
  Controle de Roll : Subsystem
  Controle de Yaw : Subsystem
  Out1 : Outport
  Out2 : Outport  Port=2
  Out3 : Outport  Port=3
  wires:
  In2/1 -> Controle de Roll/2(phi)  "phi"
  In4/1 -> Controle de Pitch/1(theta_ref)  "theta_ref"
  In3/1 -> Controle de Roll/3(P)  "P"
  In1/1 -> Controle de Roll/1(phi_ref)  "phi_ref"
  Controle de Roll/1(U_roll) -> Out1/1  "U_L"
  Controle de Pitch/1(U_pitch) -> Out2/1  "U_M"
  Controle de Yaw/1(U_yaw) -> Out3/1  "U_N"
  In5/1 -> Controle de Pitch/2(theta)  "theta"
  In6/1 -> Controle de Pitch/3(Q)  "Q"
  In7/1 -> Controle de Yaw/1(psi_ref)  "psi_ref"
  In8/1 -> Controle de Yaw/2(psi)  "psi"
  In9/1 -> Controle de Yaw/3(R)  "R"

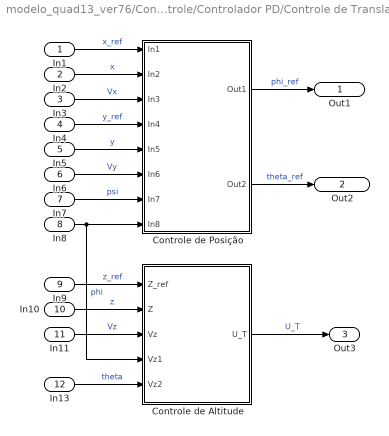
== system modelo_quad13_ver76/Controle/Controlador PD/Controle de Translação ==
  In1 : Inport
  In2 : Inport  Port=2
  In3 : Inport  Port=3
  In4 : Inport  Port=4
  In5 : Inport  Port=5
  In6 : Inport  Port=6
  In7 : Inport  Port=7
  In8 : Inport  Port=8
  In9 : Inport  Port=9
  In10 : Inport  Port=10
  In11 : Inport  Port=11
  In13 : Inport  Port=12
  Controle de Altitude : Subsystem
  Controle de Posição : Subsystem
  Out1 : Outport
  Out2 : Outport  Port=2
  Out3 : Outport  Port=3
  wires:
  Controle de Altitude/1(U_T) -> Out3/1  "U_T"
  Controle de Posição/1(Out1) -> Out1/1  "phi_ref"
  Controle de Posição/2(Out2) -> Out2/1  "theta_ref"
  In1/1 -> Controle de Posição/1(In1)  "x_ref"
  In2/1 -> Controle de Posição/2(In2)  "x"
  In3/1 -> Controle de Posição/3(In3)  "Vx"
  In4/1 -> Controle de Posição/4(In4)  "y_ref"
  In5/1 -> Controle de Posição/5(In5)  "y"
  In6/1 -> Controle de Posição/6(In6)  "Vy"
  In7/1 -> Controle de Posição/7(In7)  "psi"
  In9/1 -> Controle de Altitude/1(Z_ref)  "z_ref"
  In10/1 -> Controle de Altitude/2(Z)  "z"
  In11/1 -> Controle de Altitude/3(Vz)  "Vz"
  In8/1 -> Controle de Altitude/4(Vz1), Controle de Posição/8(In8)  "phi"
  In13/1 -> Controle de Altitude/5(Vz2)  "theta"

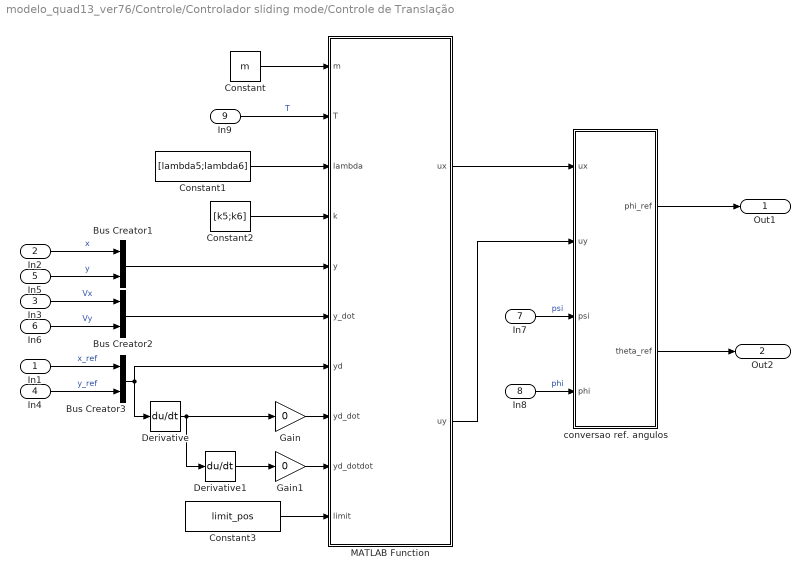
== system modelo_quad13_ver76/Controle/Controlador sliding mode/Controle de Translação ==
  In1 : Inport
  In2 : Inport  Port=2
  In3 : Inport  Port=3
  In4 : Inport  Port=4
  In5 : Inport  Port=5
  In6 : Inport  Port=6
  In7 : Inport  Port=7
  In8 : Inport  Port=8
  In9 : Inport  Port=9
  Bus Creator1 : BusCreator  Inputs=2
  Bus Creator2 : BusCreator  Inputs=2
  Bus Creator3 : BusCreator  Inputs=2
  Constant : Constant  Value=m
  Constant1 : Constant  Value=[lambda5;lambda6]
  Constant2 : Constant  Value=[k5;k6]
  Constant3 : Constant  Value=limit_pos
  Derivative : Derivative
  Derivative1 : Derivative
  Gain : Gain  Gain=0
  Gain1 : Gain  Gain=0
  MATLAB Function : MATLAB Function  TreatAsAtomicUnit=on
  conversao ref. angulos : MATLAB Function  TreatAsAtomicUnit=on
  Out1 : Outport
  Out2 : Outport  Port=2
  wires:
  MATLAB Function/1(ux) -> conversao ref. angulos/1(ux)
  conversao ref. angulos/1(phi_ref) -> Out1/1
  conversao ref. angulos/2(theta_ref) -> Out2/1
  Constant/1 -> MATLAB Function/1(m)
  Constant1/1 -> MATLAB Function/3(lambda)
  Constant2/1 -> MATLAB Function/4(k)
  Bus Creator1/1 -> MATLAB Function/5(y)
  In2/1 -> Bus Creator1/1  "x"
  In5/1 -> Bus Creator1/2  "y"
  Bus Creator2/1 -> MATLAB Function/6(y_dot)
  In3/1 -> Bus Creator2/1  "Vx"
  In6/1 -> Bus Creator2/2  "Vy"
  Bus Creator3/1 -> MATLAB Function/7(yd), Derivative/1
  In1/1 -> Bus Creator3/1  "x_ref"
  In4/1 -> Bus Creator3/2  "y_ref"
  Derivative/1 -> Gain/1, Derivative1/1
  Derivative1/1 -> Gain1/1
  In7/1 -> conversao ref. angulos/3(psi)  "psi"
  In8/1 -> conversao ref. angulos/4(phi)  "phi"
  Gain/1 -> MATLAB Function/8(yd_dot)
  Gain1/1 -> MATLAB Function/9(yd_dotdot)
  In9/1 -> MATLAB Function/2(T)  "T"
  Constant3/1 -> MATLAB Function/10(limit)
  MATLAB Function/2(uy) -> conversao ref. angulos/2(uy)

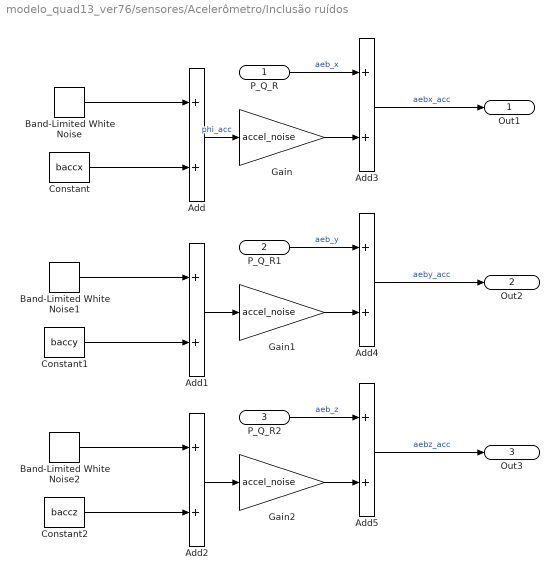
== system modelo_quad13_ver76/sensores/Acelerômetro/Inclusão ruídos ==
  P_Q_R : Inport
  P_Q_R1 : Inport  Port=2
  P_Q_R2 : Inport  Port=3
  Add{,1..5} (6 alike) : Sum
  Band-Limited White Noise : simulink/Sources/Band-Limited White Noise  Cov=varAccx  Ts=Tsr  seed=[23341]
  Band-Limited White Noise1 : simulink/Sources/Band-Limited White Noise  Cov=varAccy  Ts=Tsr  seed=[23341]
  Band-Limited White Noise2 : simulink/Sources/Band-Limited White Noise  Cov=varAccy  Ts=Tsr  seed=[23341]
  Constant : Constant  Value=baccx
  Constant1 : Constant  Value=baccy
  Constant2 : Constant  Value=baccz
  Gain : Gain  Gain=accel_noise
  Gain1 : Gain  Gain=accel_noise
  Gain2 : Gain  Gain=accel_noise
  Out1 : Outport
  Out2 : Outport  Port=2
  Out3 : Outport  Port=3
  wires:
  Band-Limited White Noise/1 -> Add/1
  Constant/1 -> Add/2
  Band-Limited White Noise1/1 -> Add1/1
  Add3/1 -> Out1/1  "aebx_acc"
  P_Q_R/1 -> Add3/1  "aeb_x"
  Add/1 -> Gain/1  "phi_acc"
  Gain/1 -> Add3/2
  Constant1/1 -> Add1/2
  Add1/1 -> Gain1/1
  Gain1/1 -> Add4/2
  P_Q_R1/1 -> Add4/1  "aeb_y"
  Add4/1 -> Out2/1  "aeby_acc"
  Band-Limited White Noise2/1 -> Add2/1
  Constant2/1 -> Add2/2
  Add2/1 -> Gain2/1
  Gain2/1 -> Add5/2
  P_Q_R2/1 -> Add5/1  "aeb_z"
  Add5/1 -> Out3/1  "aebz_acc"

== system modelo_quad13_ver76/sensores/GPS/GPS_LAT ==
  north_Disp_m : Inport
  Band-Limited White Noise : simulink/Sources/Band-Limited White Noise  Cov=var_disp_gps  Ts=Tnoise_gps  seed=[9941]
  Sum : Sum  Inputs=|++
  Zero-Order Hold : ZeroOrderHold  SampleTime=TsGPS
  gps_noise_on : Gain  Gain=gps_noise_on
  xn_gps : Outport
  wires:
  Sum/1 -> Zero-Order Hold/1
  north_Disp_m/1 -> Sum/1
  Zero-Order Hold/1 -> xn_gps/1
  Band-Limited White Noise/1 -> gps_noise_on/1
  gps_noise_on/1 -> Sum/2

== system modelo_quad13_ver76/sensores/GPS/GPS_LON ==
  east_Disp_m : Inport
  Band-Limited White Noise : simulink/Sources/Band-Limited White Noise  Cov=var_disp_gps  Ts=Tnoise_gps  seed=[334421]
  Sum : Sum  Inputs=|++
  Zero-Order Hold : ZeroOrderHold  SampleTime=TsGPS
  gps_noise_on : Gain  Gain=gps_noise_on
  ye_gps : Outport
  wires:
  Sum/1 -> Zero-Order Hold/1
  east_Disp_m/1 -> Sum/1
  Zero-Order Hold/1 -> ye_gps/1
  Band-Limited White Noise/1 -> gps_noise_on/1
  gps_noise_on/1 -> Sum/2

== system modelo_quad13_ver76/sensores/GPS/GPS_VEL ==
  north_Speed_mps : Inport
  Band-Limited White Noise : simulink/Sources/Band-Limited White Noise  Cov=var_vel_gps  Ts=Tnoise_gps  seed=[991141]
  First-Order Hold : simulink/Discrete/First-Order Hold  DisableCoverage=on  Ts=TsGPS
  Sum : Sum  Inputs=|++
  Zero-Order Hold : ZeroOrderHold  SampleTime=TsGPS
  gps_noise_on : Gain  Gain=gps_noise_on
  north_Speed_GPS_mps : Outport
  wires:
  Sum/1 -> First-Order Hold/1
  north_Speed_mps/1 -> Sum/1
  First-Order Hold/1 -> north_Speed_GPS_mps/1
  Band-Limited White Noise/1 -> gps_noise_on/1
  gps_noise_on/1 -> Sum/2

== system modelo_quad13_ver76/sensores/GPS/GPS_VEL1 ==
  east_Speed_mps : Inport
  Band-Limited White Noise : simulink/Sources/Band-Limited White Noise  Cov=var_vel_gps  Ts=Tnoise_gps  seed=[994551]
  First-Order Hold : simulink/Discrete/First-Order Hold  DisableCoverage=on  Ts=TsGPS
  Sum : Sum  Inputs=|++
  gps_noise_on : Gain  Gain=gps_noise_on
  east_Speed_GPS_mps : Outport
  wires:
  Sum/1 -> First-Order Hold/1
  east_Speed_mps/1 -> Sum/1
  First-Order Hold/1 -> east_Speed_GPS_mps/1
  Band-Limited White Noise/1 -> gps_noise_on/1
  gps_noise_on/1 -> Sum/2

== system modelo_quad13_ver76/sensores/GPS/GPS_VEL2 ==
  down_Speed_mps : Inport
  Band-Limited White Noise : simulink/Sources/Band-Limited White Noise  Cov=var_vel_gps  Ts=Tnoise_gps  seed=[997741]
  First-Order Hold : simulink/Discrete/First-Order Hold  DisableCoverage=on  Ts=TsGPS
  Sum : Sum  Inputs=|++
  gps_noise_on : Gain  Gain=gps_noise_on
  down_Speed_GPS_mps : Outport
  wires:
  Sum/1 -> First-Order Hold/1
  down_Speed_mps/1 -> Sum/1
  First-Order Hold/1 -> down_Speed_GPS_mps/1
  Band-Limited White Noise/1 -> gps_noise_on/1
  gps_noise_on/1 -> Sum/2

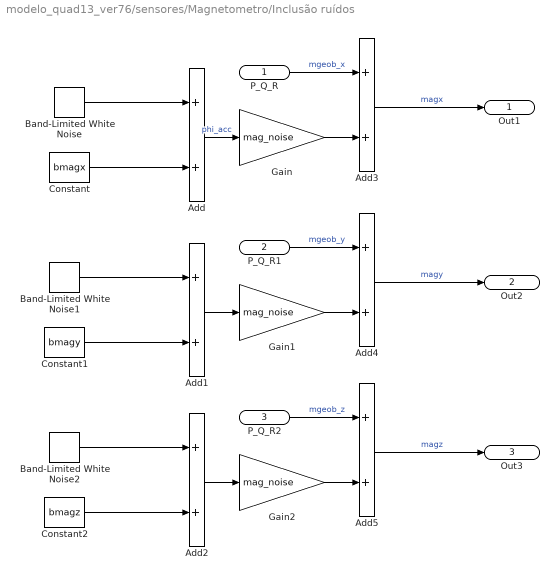
== system modelo_quad13_ver76/sensores/Magnetometro/Inclusão ruídos ==
  P_Q_R : Inport
  P_Q_R1 : Inport  Port=2
  P_Q_R2 : Inport  Port=3
  Add{,1..5} (6 alike) : Sum
  Band-Limited White Noise : simulink/Sources/Band-Limited White Noise  Cov=varMagx  Ts=Tsr  seed=[23341]
  Band-Limited White Noise1 : simulink/Sources/Band-Limited White Noise  Cov=varMagy  Ts=Tsr  seed=[23341]
  Band-Limited White Noise2 : simulink/Sources/Band-Limited White Noise  Cov=varMagy  Ts=Tsr  seed=[23341]
  Constant : Constant  Value=bmagx
  Constant1 : Constant  Value=bmagy
  Constant2 : Constant  Value=bmagz
  Gain : Gain  Gain=mag_noise
  Gain1 : Gain  Gain=mag_noise
  Gain2 : Gain  Gain=mag_noise
  Out1 : Outport
  Out2 : Outport  Port=2
  Out3 : Outport  Port=3
  wires:
  Band-Limited White Noise/1 -> Add/1
  Constant/1 -> Add/2
  Band-Limited White Noise1/1 -> Add1/1
  Add3/1 -> Out1/1  "magx"
  P_Q_R/1 -> Add3/1  "mgeob_x"
  Add/1 -> Gain/1  "phi_acc"
  Gain/1 -> Add3/2
  Constant1/1 -> Add1/2
  Add1/1 -> Gain1/1
  Gain1/1 -> Add4/2
  P_Q_R1/1 -> Add4/1  "mgeob_y"
  Add4/1 -> Out2/1  "magy"
  Band-Limited White Noise2/1 -> Add2/1
  Constant2/1 -> Add2/2
  Add2/1 -> Gain2/1
  Gain2/1 -> Add5/2
  P_Q_R2/1 -> Add5/1  "mgeob_z"
  Add5/1 -> Out3/1  "magz"

== system modelo_quad13_ver76/sensores/aceleracao_inercial/Modulus ==
  In1 : Inport
  Dot Product : DotProduct  InputSameDT=on  OutDataTypeStr=Inherit: Inherit via internal rule
  Sqrt : Sqrt  SaturateOnIntegerOverflow=on
  Out1 : Outport
  wires:
  In1/1 -> Dot Product/2, Dot Product/1
  Dot Product/1 -> Sqrt/1
  Sqrt/1 -> Out1/1

== system modelo_quad13_ver76/Controle/Controlador PD/Controle de Rotação/Controle de Pitch ==
  theta_ref : Inport
  theta : Inport  Port=2
  Q : Inport  Port=3
  Gain : Gain  Gain=Pitch_P
  Gain1 : Gain  Gain=-Pitch_D
  Scope3 : Scope
      settings: YMin=37.75  YMax=40  SaveName=ScopeData3
  Sum : Sum  Inputs=|+-
  Sum1 : Sum  Inputs=|++
  U_pitch : Outport
  wires:
  Sum/1 -> Gain/1
  theta_ref/1 -> Sum/1  "theta_ref"
  Sum1/1 -> Scope3/1, U_pitch/1
  Gain/1 -> Sum1/1
  theta/1 -> Sum/2
  Gain1/1 -> Sum1/2
  Q/1 -> Gain1/1

== system modelo_quad13_ver76/Controle/Controlador PD/Controle de Rotação/Controle de Roll ==
  phi_ref : Inport
  phi : Inport  Port=2
  P : Inport  Port=3
  Gain : Gain  Gain=Roll_P
  Gain1 : Gain  Gain=-Roll_D
  Scope3 : Scope
      settings: YMin=-2500  YMax=2500  SaveName=ScopeData3
  Sum : Sum  Inputs=|+-
  Sum1 : Sum  Inputs=|++
  U_roll : Outport
  wires:
  Sum/1 -> Gain/1
  P/1 -> Gain1/1
  Gain/1 -> Sum1/1
  Gain1/1 -> Sum1/2
  Sum1/1 -> Scope3/1, U_roll/1
  phi_ref/1 -> Sum/1  "phi_ref"
  phi/1 -> Sum/2

== system modelo_quad13_ver76/Controle/Controlador PD/Controle de Rotação/Controle de Yaw ==
  psi_ref : Inport
  psi : Inport  Port=2
  R : Inport  Port=3
  Gain : Gain  Gain=Yaw_P
  Gain1 : Gain  Gain=-Yaw_D
  Scope3 : Scope
      settings: YMin=37.75  YMax=40  SaveName=ScopeData3
  Sum : Sum  Inputs=|+-
  Sum1 : Sum  Inputs=|++
  U_yaw : Outport
  wires:
  Sum/1 -> Gain/1
  Sum1/1 -> Scope3/1, U_yaw/1
  psi/1 -> Sum/2
  psi_ref/1 -> Sum/1  "psi_ref"
  Gain/1 -> Sum1/1
  R/1 -> Gain1/1
  Gain1/1 -> Sum1/2

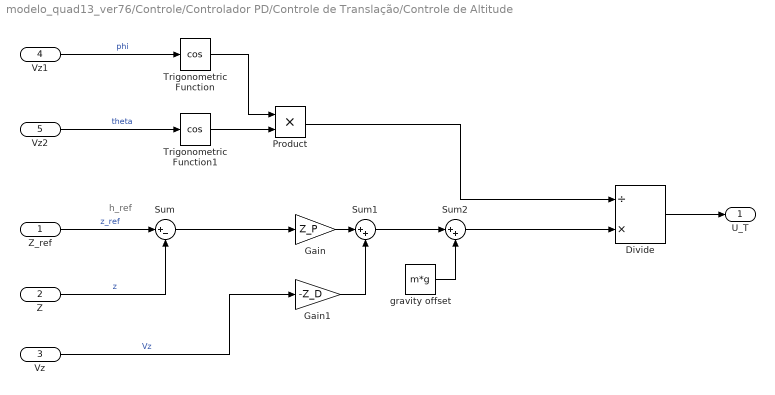
== system modelo_quad13_ver76/Controle/Controlador PD/Controle de Translação/Controle de Altitude ==
  note: h_ref
  Z_ref : Inport
  Z : Inport  Port=2
  Vz : Inport  Port=3
  Vz1 : Inport  Port=4
  Vz2 : Inport  Port=5
  Divide : Product  Inputs=/*
  Gain : Gain  Gain=Z_P
  Gain1 : Gain  Gain=-Z_D
  Product : Product
  Sum : Sum  Inputs=|+-
  Sum1 : Sum  Inputs=|++
  Sum2 : Sum  Inputs=|++
  Trigonometric Function : Trigonometry  Operator=cos
  Trigonometric Function1 : Trigonometry  Operator=cos
  gravity offset : Constant  Value=m*g
  U_T : Outport
  wires:
  Sum/1 -> Gain/1
  Sum2/1 -> Divide/2
  Vz/1 -> Gain1/1  "Vz"
  gravity offset/1 -> Sum2/2
  Z_ref/1 -> Sum/1  "z_ref"
  Z/1 -> Sum/2  "z"
  Gain/1 -> Sum1/1
  Gain1/1 -> Sum1/2
  Sum1/1 -> Sum2/1
  Trigonometric Function1/1 -> Product/2
  Trigonometric Function/1 -> Product/1
  Product/1 -> Divide/1
  Divide/1 -> U_T/1
  Vz1/1 -> Trigonometric Function/1  "phi"
  Vz2/1 -> Trigonometric Function1/1  "theta"

== system modelo_quad13_ver76/Controle/Controlador PD/Controle de Translação/Controle de Posição ==
  In1 : Inport
  In2 : Inport  Port=2
  In3 : Inport  Port=3
  In4 : Inport  Port=4
  In5 : Inport  Port=5
  In6 : Inport  Port=6
  In7 : Inport  Port=7
  In8 : Inport  Port=8
  Controle de Posição x : Subsystem
  Controle de Posição y : Subsystem
  Gain1 : Gain  Gain=controle
  Gain2 : Gain  Gain=controle
  conversao ref. angulos : MATLAB Function  TreatAsAtomicUnit=on
  Out1 : Outport
  Out2 : Outport  Port=2
  wires:
  In1/1 -> Controle de Posição x/1(phi_ref)  "x_ref"
  In5/1 -> Controle de Posição y/2(phi)  "y"
  In2/1 -> Controle de Posição x/2(phi)  "x"
  In4/1 -> Controle de Posição y/1(phi_ref)  "y_ref"
  In6/1 -> Controle de Posição y/3(P)  "Vy"
  In3/1 -> Controle de Posição x/3(P)  "Vx"
  conversao ref. angulos/1(phi_ref) -> Gain1/1  "phi_ref"
  conversao ref. angulos/2(theta_ref) -> Gain2/1  "theta_ref"
  Controle de Posição x/1(Ux) -> conversao ref. angulos/1(ux)
  Controle de Posição y/1(Ux) -> conversao ref. angulos/2(uy)
  In7/1 -> conversao ref. angulos/3(psi)  "psi"
  In8/1 -> conversao ref. angulos/4(phi)  "phi"
  Gain1/1 -> Out1/1  "phi_ref"
  Gain2/1 -> Out2/1  "theta_ref"

== system modelo_quad13_ver76/Controle/Controlador PD/Controle de Translação/Controle de Posição/Controle de Posição x ==
  phi_ref : Inport
  phi : Inport  Port=2
  P : Inport  Port=3
  Gain : Gain  Gain=pos_P
  Gain1 : Gain  Gain=-pos_D
  Gain2 : Gain  Gain=controle
  Sum : Sum  Inputs=|+-
  Sum1 : Sum  Inputs=|++
  Ux : Outport
  wires:
  Sum/1 -> Gain/1
  P/1 -> Gain1/1  "Vx"
  Gain/1 -> Sum1/1
  Gain1/1 -> Sum1/2
  Sum1/1 -> Gain2/1  "Ux"
  phi_ref/1 -> Sum/1  "x_ref"
  phi/1 -> Sum/2  "x"
  Gain2/1 -> Ux/1

== system modelo_quad13_ver76/Controle/Controlador PD/Controle de Translação/Controle de Posição/Controle de Posição y ==
  phi_ref : Inport
  phi : Inport  Port=2
  P : Inport  Port=3
  Gain : Gain  Gain=pos_P
  Gain1 : Gain  Gain=-pos_D
  Gain2 : Gain  Gain=controle
  Sum : Sum  Inputs=|+-
  Sum1 : Sum  Inputs=|++
  Ux : Outport
  wires:
  Sum/1 -> Gain/1
  P/1 -> Gain1/1  "Vy"
  Gain/1 -> Sum1/1
  Gain1/1 -> Sum1/2
  Sum1/1 -> Gain2/1  "Uy"
  phi_ref/1 -> Sum/1  "y_ref"
  phi/1 -> Sum/2  "y"
  Gain2/1 -> Ux/1

== matlab function Dinâmica do quadricoptero/MATLAB Function ==
  data: Vel_dot output double; Ang_dot output double; w1 input double; w2 input double; w3 input double; w4 input double; J input double; g input double; ct input double; cq input double; d input double; m input double; V_Ang_dot output double; Ang input double; V_Ang input double; aeb output double; mgeob output double size=[3,1]; mgeo input double size=[3,1]
function [Vel_dot,Ang_dot,V_Ang_dot, aeb, mgeob] = quad_model(w1,w2,w3,w4,J,g,ct,cq,d,m,Ang,V_Ang,mgeo)


Jxx=J(1);
Jyy=J(2);
Jzz=J(3);
Jm=J(4);

phi = Ang(1);
theta = Ang(2);
psi = Ang(3);

P = V_Ang(1);
Q = V_Ang(2);
R = V_Ang(3);

%derivadas ângulos de euler
pqr2euler = [1, tan(theta)*sin(phi), tan(theta)*cos(phi);
             0, cos(phi), -sin(phi);
             0, sin(phi)/cos(theta), cos(phi)/cos(theta)];

Ang_dot = pqr2euler*V_Ang;

%acelerações de translação
T = ct*(w1^2+w2^2+w3^2+w4^2);

Rot_b_e=[cos(psi)*cos(theta), cos(psi)*sin(phi)*sin(theta)-cos(phi)*sin(psi), sin(phi)*sin(psi)+cos(phi)*cos(psi)*sin(theta);
         cos(theta)*sin(psi), cos(phi)*cos(psi)+sin(phi)*sin(psi)*sin(theta), cos(phi)*sin(psi)*sin(theta)-cos(psi)*sin(phi);
         -sin(theta), cos(theta)*sin(phi), cos(phi)*cos(theta)];

Vel_dot = [0;0;g]+(1/m)*Rot_b_e*[0;0;-T];

%aceleração específica no sistema de referência do corpo
 aeb=Rot_b_e'*(Vel_dot-[0;0;g]); % ERRO -> Tem que converter a gravidade para o sistema do corpo
%aeb=Rot_b_e'*(-[0;0;g]);

% Campo magnetico terrestre no sistema de referencia do corpo
mgeob=Rot_b_e'*mgeo;

%acelerações angulares
L = d*ct*(w4^2-w2^2);
M = d*ct*(w1^2-w3^2);
N = cq*(w1^2-w2^2+w3^2-w4^2);

tgir_x = Jm*Q*(-w1^2+w2^2-w3^2+w4^2);
tgir_y = Jm*P*(w1^2-w2^2+w3^2-w4^2);

V_Ang_dot=[(1/Jxx)*(L+tgir_x-Q*R*(Jzz-Jyy));
        (1/Jyy)*(M+tgir_y-P*R*(Jxx-Jzz));
        (1/Jzz)*(N-P*Q*(Jyy-Jxx))];

== matlab function Conversão dos comandos/MATLAB Function ==
  data: u_T input double; w1d output double; u_L input double; u_M input double; u_N input double; w2d output double; w3d output double; w4d output double; d input double; ct input double; cq input double
function [w1d,w2d,w3d,w4d] = commands_conv(u_T,u_L,u_M,u_N,d,ct,cq)


u_z = u_T/(4*ct);
u_phi = u_L/(2*d*ct);
u_theta = u_M/(2*d*ct);
u_psi = u_N/(4*cq);

w1d_sq=u_z+u_theta+u_psi;
w2d_sq=u_z-u_phi-u_psi;
w3d_sq=u_z-u_theta+u_psi;
w4d_sq=u_z+u_phi-u_psi;


if w1d_sq<0
    w1d_sq=0;
end
if w2d_sq<0
    w2d_sq=0;
end
if w3d_sq<0
    w3d_sq=0;
end
if w4d_sq<0
    w4d_sq=0;
end



w1d = sqrt(w1d_sq);
w2d = sqrt(w2d_sq);
w3d = sqrt(w3d_sq);
w4d = sqrt(w4d_sq);

== matlab function Motores/Motor 1/MATLAB Function ==
  data: wd input double; w input double; ke input double; cq input double; kt input double; R input double; Ja input double; wder output double
function wder = motor(wd,w,ke,cq,kt,R,Ja)

wss = wd;

V = ke*wss + (cq*R/kt)*wss^2;

wder = -(kt*ke*w)/(R*Ja) - (cq*w^2/Ja) + (kt*V)/(Ja*R);

== matlab function Motores/Motor 2/MATLAB Function ==
  data: wd input double; w input double; ke input double; cq input double; kt input double; R input double; Ja input double; wder output double
function wder = motor(wd,w,ke,cq,kt,R,Ja)

wss = wd;

V = ke*wss + (cq*R/kt)*wss^2;

wder = -(kt*ke*w)/(R*Ja) - (cq*w^2/Ja) + (kt*V)/(Ja*R);

== matlab function Motores/Motor 3/MATLAB Function ==
  data: wd input double; w input double; ke input double; cq input double; kt input double; R input double; Ja input double; wder output double
function wder = motor(wd,w,ke,cq,kt,R,Ja)

wss = wd;

V = ke*wss + (cq*R/kt)*wss^2;

wder = -(kt*ke*w)/(R*Ja) - (cq*w^2/Ja) + (kt*V)/(Ja*R);

== matlab function Motores/Motor 4/MATLAB Function ==
  data: wd input double; w input double; ke input double; cq input double; kt input double; R input double; Ja input double; wder output double
function wder = motor(wd,w,ke,cq,kt,R,Ja)

wss = wd;

V = ke*wss + (cq*R/kt)*wss^2;

wder = -(kt*ke*w)/(R*Ja) - (cq*w^2/Ja) + (kt*V)/(Ja*R);
